simulink model "project1_simulink"  (R2019a)
settings: Solver=FixedStepDiscrete  StartTime=0.0  StopTime=0.05  FixedStep=Ts  MaxStep=1e-4  RelTol=1e-3
libraries: powerlib x26
settings Model: Creator=nquintan  LastModifiedBy=tolugben
settings DataIOCC: ReturnWorkspaceOutputs=off
settings DebuggingCC: ArithmeticOperatorsInVariantConditions=warning
settings SFSimCC: SimUseLocalCustomCode=off
settings RTWCC: RTWUseLocalCustomCode=off
settings CodeAppCC: StateflowObjectComments=on
settings SimscapeCC: SimscapeNormalizeSystem=off

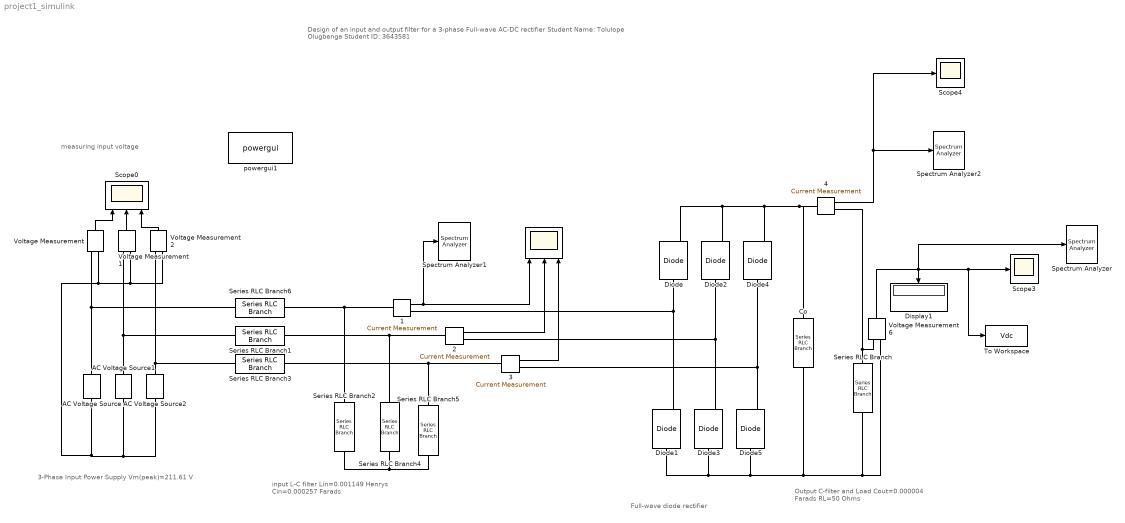
== system project1_simulink ==
  note: 3-Phase Input Power Supply
      | Vm(peak)=211.61 V
  note: Design of an input and output filter for a 3-phase Full-wave AC-DC rectifier
      |
      | Student Name: Tolulope Olugbenga
      | Student ID: 3643581
  note: measuring input voltage
  note: input L-C filter
      | Lin=0.001149 Henrys
      | Cin=0.000257 Farads
  note: Full-wave diode rectifier
  note: Output C-filter and Load
      | Cout=0.000004 Farads
      | RL=50 Ohms
   {1..4} (4 alike) : powerlib/Measurements/Current Measurement  PhasorSimulation=off  OutputType=Complex  PSBequivalent=0
      settings: SourceProductName=Simscape Electrical
  " " : Scope  NumInputPorts=3
  AC Voltage Source : powerlib/Electrical Sources/AC Voltage Source  Amplitude=211.6099  Phase=0  Frequency=60  SampleTime=0  Measurements=None  BusType=swing  Pref=10e3  Qref=0  Qmin=-inf  Qmax=+inf
      settings: SourceProductName=Simscape Electrical
  AC Voltage Source1 : powerlib/Electrical Sources/AC Voltage Source  Amplitude=211.6099  Phase=120  Frequency=60  SampleTime=0  Measurements=None  BusType=swing  Pref=10e3  Qref=0  Qmin=-inf  Qmax=+inf
      settings: SourceProductName=Simscape Electrical
  AC Voltage Source2 : powerlib/Electrical Sources/AC Voltage Source  Amplitude=211.6099  Phase=240  Frequency=60  SampleTime=0  Measurements=None  BusType=swing  Pref=10e3  Qref=0  Qmin=-inf  Qmax=+inf
      settings: SourceProductName=Simscape Electrical
  Co : powerlib/Elements/Series RLC Branch  LConnTagsString=__new0  RConnTagsString=__new0  BranchType=C  Resistance=1  Inductance=1e-3  SetiL0=off  InitialCurrent=0  Capacitance=0.000004  Setx0=off  InitialVoltage=0  Measurements=None
      settings: SourceProductName=Simscape Electrical
  Diode{,1..5} (6 alike) : powerlib/Power Electronics/Diode  Ron=0.001  Lon=0  Vf=0.8  IC=0  UseSnubber=off  Rs=500  Cs=250e-9  Measurements=on
      settings: SourceProductName=Simscape Electrical
  Display1 : Display
  Scope0 : Scope  NumInputPorts=3
  Scope3 : Scope
  "Scope4 " : Scope
  Series RLC Branch : powerlib/Elements/Series RLC Branch  LConnTagsString=__new0  RConnTagsString=__new0  BranchType=R  Resistance=50  Inductance=1e-3  SetiL0=off  InitialCurrent=0  Capacitance=1e-6  Setx0=off  InitialVoltage=0  Measurements=None
      settings: SourceProductName=Simscape Electrical
  Series RLC Branch1 : powerlib/Elements/Series RLC Branch  LConnTagsString=__new0  RConnTagsString=__new0  BranchType=L  Resistance=1  Inductance=0.001149  SetiL0=off  InitialCurrent=0  Capacitance=1e-6  Setx0=off  InitialVoltage=0  Measurements=None
      settings: SourceProductName=Simscape Electrical
  Series RLC Branch2 : powerlib/Elements/Series RLC Branch  LConnTagsString=__new0  RConnTagsString=__new0  BranchType=C  Resistance=1  Inductance=1e-3  SetiL0=off  InitialCurrent=0  Capacitance=0.000257  Setx0=off  InitialVoltage=0  Measurements=None
      settings: SourceProductName=Simscape Electrical
  Series RLC Branch3 : powerlib/Elements/Series RLC Branch  LConnTagsString=__new0  RConnTagsString=__new0  BranchType=L  Resistance=1  Inductance=0.001149  SetiL0=off  InitialCurrent=0  Capacitance=1e-6  Setx0=off  InitialVoltage=0  Measurements=None
      settings: SourceProductName=Simscape Electrical
  Series RLC Branch4 : powerlib/Elements/Series RLC Branch  LConnTagsString=__new0  RConnTagsString=__new0  BranchType=C  Resistance=1  Inductance=1e-3  SetiL0=off  InitialCurrent=0  Capacitance=0.000257  Setx0=off  InitialVoltage=0  Measurements=None
      settings: SourceProductName=Simscape Electrical
  Series RLC Branch5 : powerlib/Elements/Series RLC Branch  LConnTagsString=__new0  RConnTagsString=__new0  BranchType=C  Resistance=1  Inductance=1e-3  SetiL0=off  InitialCurrent=0  Capacitance=0.000257  Setx0=off  InitialVoltage=0  Measurements=None
      settings: SourceProductName=Simscape Electrical
  Series RLC Branch6 : powerlib/Elements/Series RLC Branch  LConnTagsString=__new0  RConnTagsString=__new0  BranchType=L  Resistance=1  Inductance=0.001149  SetiL0=off  InitialCurrent=0  Capacitance=1e-6  Setx0=off  InitialVoltage=0  Measurements=None
      settings: SourceProductName=Simscape Electrical
  Spectrum Analyzer : SpectrumAnalyzer
  Spectrum Analyzer1 : SpectrumAnalyzer
  Spectrum Analyzer2 : SpectrumAnalyzer
  To Workspace : ToWorkspace  VariableName=Vdc  SaveFormat=Structure With Time  SampleTime=-1
  Voltage Measurement{,1..2,6} (4 alike) : powerlib/Measurements/Voltage Measurement  PhasorSimulation=off  OutputType=Complex  PSBequivalent=0
      settings: SourceProductName=Simscape Electrical
  powergui1 : powerlib/powergui  Priority=1  SimulationMode=Discrete  SampleTime=1e-5  frequency=60  Iterations=50  frequencyindice=60  Pbase=100e6  ErrMax=1e-4  UnitsV=kV  UnitsW=MW  buscounter=0  FunctionMessages=off  echomessages=off  EnableUseOfTLC=off  CurrentSourceSwitches=off  DisableSnubberDevices=off  DisableRonSwitches=off  DisableVfSwitches=off  DisplayEquations=off  AutomaticDiscreteSolvers=off  SolverType=Tustin  Interpol=off  ExternalGateDelay=off  methode=off  Ts=0  x0status=blocks  SPID=off  SwTol=0  HookPort=off  NonlinearTolerance=0  nMaxIteration=15  ContinueOnMaxIteration=off  RestoreLinks=warning  ResistiveCurrentMeasurement=off  Frange=[0:2:500]  Ylog=off  Xlog=on  ShowGrid=off  save=off  variable=ZData  structure=Aa  ZoomFFT=off  StartTime=0.0  cycles=1  DisplayStyle=4  fundamental=60  FreqAxis=off  MaxFrequency=1000  frequencyindicesteady=1  RmsSteady=1  display=off
      settings: SourceProductName=Simscape Electrical
  wires:
  Voltage Measurement/1 -> Scope0/1
  Voltage Measurement1/1 -> Scope0/2
  Voltage Measurement2/1 -> Scope0/3
  " 1"/1 -> Spectrum Analyzer1/1, " "/1
  " 2"/1 -> " "/2
  " 3"/1 -> " "/3
  " 4"/1 -> "Scope4 "/1, Spectrum Analyzer2/1
  Voltage Measurement6/1 -> Spectrum Analyzer/1, To Workspace/1, Scope3/1, Display1/1
  connections:
  AC Voltage Source/LConn1 -- Voltage Measurement2/LConn2 -- Voltage Measurement1/LConn2 -- Voltage Measurement/LConn2 -- AC Voltage Source2/LConn1 -- AC Voltage Source1/LConn1
  Voltage Measurement/LConn1 -- AC Voltage Source/RConn1 -- Series RLC Branch6/LConn1
  Voltage Measurement1/LConn1 -- AC Voltage Source1/RConn1 -- Series RLC Branch1/LConn1
  Voltage Measurement2/LConn1 -- Series RLC Branch3/LConn1 -- AC Voltage Source2/RConn1
  Series RLC Branch/LConn1 -- " 4"/RConn1 -- Voltage Measurement6/LConn1
  Voltage Measurement6/LConn2 -- Diode3/LConn1 -- Diode1/LConn1 -- Diode5/LConn1 -- Co/RConn1 -- Series RLC Branch/RConn1
  Diode1/RConn1 -- " 1"/RConn1 -- Diode/LConn1
  Series RLC Branch1/RConn1 -- " 2"/LConn1 -- Series RLC Branch4/LConn1
  Diode4/LConn1 -- Diode5/RConn1 -- " 3"/RConn1
  Series RLC Branch2/RConn1 -- Series RLC Branch5/RConn1 -- Series RLC Branch4/RConn1
  Series RLC Branch5/LConn1 -- " 3"/LConn1 -- Series RLC Branch3/RConn1
  Diode2/LConn1 -- " 2"/RConn1 -- Diode3/RConn1
  Series RLC Branch2/LConn1 -- Series RLC Branch6/RConn1 -- " 1"/LConn1
  Diode/RConn1 -- " 4"/LConn1 -- Co/LConn1 -- Diode4/RConn1 -- Diode2/RConn1
